simulink model "controller_ballcatcher"  (R2018b)
settings: Solver=FixedStepDiscrete  StartTime=0.0  StopTime=10.0  FixedStep=timing.T_iiwa  RelTol=1e-3
InitFcn:
  | iiwa_joint_trajectoryfollowingcontrol_rigid_parameters;
values from neighbouring files (symbols this model uses):
  filter_tau_p_slow_T_1 = filter_tau_slow_T_1    [parameters.m]
  filter_tau_p_T_1 = filter_tau_T_1    [parameters.m]
  filter_tau_slow_T_1 = 1./(2*pi*[200;200;200;200;200;200;200])    [parameters.m]
  filter_tau_T_1 = 1./(2*pi*[400;400;400;400;500;1000;1000])    [parameters.m]
  filter_theta_p_slow_T_1 = filter_tau_slow_T_1    [parameters.m]
  filter_theta_p_T_1 = filter_tau_T_1    [parameters.m]
  filter_theta_slow_T_1 = filter_tau_slow_T_1    [parameters.m]
  param_nullspace = struct()    [parameters.m]
  param_robot = struct()    [parameters.m]
  sensor_torque_offset = [0.53;-0.095;-0.189;0.07;-0.058;0.0025;-0.12]    [parameters.m]
  timing = struct()    [parameters.m]
undefined symbols (not defined in the file or in its folder): param_controller
settings Model: TCT_ExtModeMexArgs=[128 131 86 77 1 1],16842784  SimulationMode=external  Creator=cha  LastModifiedBy=stefanschweng
settings SolverCC: AutoInsertRateTranBlk=on
settings DataIOCC: LoggingToFile=on  LoggingFileName=benniii.mat
settings OptimizationCC: UseFloatMulNetSlope=on  PassReuseOutputArgsThreshold=0  LocalBlockOutputs=off  EfficientFloat2IntCast=on  OptimizeBlockOrder=speed  DifferentSizesBufferReuse=on
settings DebuggingCC: ParameterTunabilityLossMsg=error
settings HardwareCC: ProdLongLongMode=on
settings ModelReferenceCC: EnableParallelModelReferenceBuilds=on  ModelReferenceNumInstancesAllowed=Single
settings SFSimCC: SimUseLocalCustomCode=off  MATLABDynamicMemAlloc=off
settings RTWCC: Description=TwinCAT Target  SystemTargetFile=TwinCAT.tlc  GenCodeOnly=on  MakeCommand=make_tct  TemplateMakefile=tct_msbuild.tmf  GenerateReport=on  RTWUseLocalCustomCode=off  TargetLang=C++
settings RTWCC: CustomHeaderCode=|
  | #define fflush(stdout)
  | #define printf(...) m_spSrv->TcReportLog(ADSLOG_MSGTYPE_LOG,__VA_ARGS__)
settings CodeAppCC: ForceParamTrailComments=on  MaxIdLength=47  OperatorAnnotations=on  StateflowObjectComments=on  MATLABSourceComments=on
settings STFCustomTargetCC: TargetLangStandard=C++03 (ISO)  CompOptLevelCompliant=on  MATLABClassNameForMDSCustomization=Simulink.SoftwareTarget.TargetSpecificTriggerConfigurationBase  GRTInterface=on  SystemTargetFile=TwinCAT.tlc

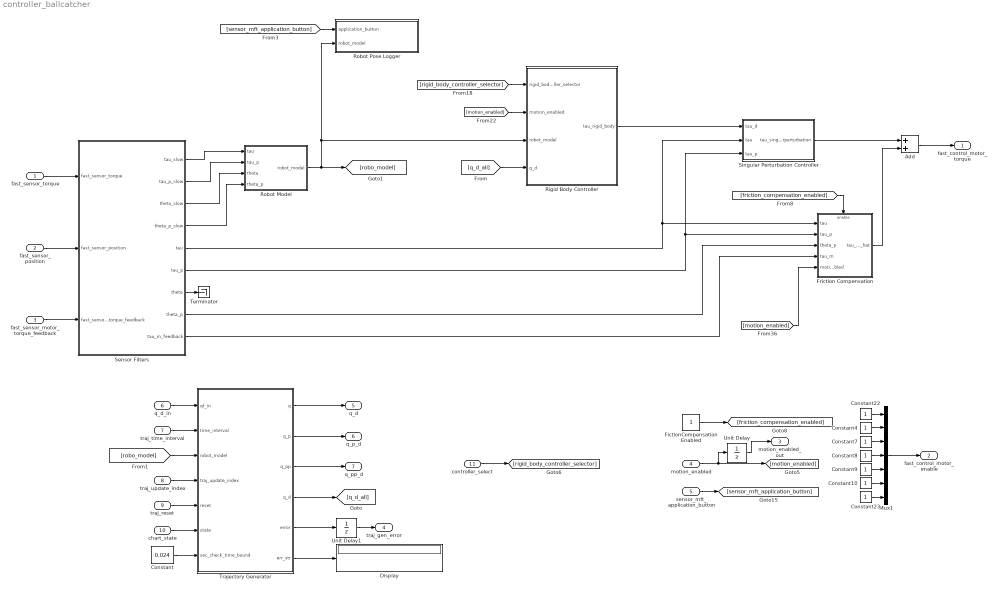
== system controller_ballcatcher ==
  fast_sensor_torque : Inport
  fast_sensor_position : Inport  Port=2
  fast_sensor_motor_torque_feedback : Inport  Port=3
  motion_enabled : Inport  Port=4
  sensor_mft_application_button : Inport  Port=5
  q_d_in : Inport  Port=6  PortDimensions=7
  traj_time_interval : Inport  Port=7  PortDimensions=2
  traj_update_index : Inport  Port=8
  traj_reset : Inport  Port=9
  chart_state : Inport  Port=10
  controller_select : Inport  Port=11
  Add : Sum
  Constant : Constant  Value=0.024
  Constant{4,7..10,22..23} (7 alike) : Constant
  Display : Display
  FictionCompensationEnabled : Constant
  Friction Compensation : Subsystem
  Mux1 : Mux  Inputs=7
  Rigid Body Controller : Subsystem
  Robot Model : MATLAB Function  TreatAsAtomicUnit=on
  Robot Pose Logger : MATLAB Function  TreatAsAtomicUnit=on
  Sensor Filters : Subsystem
  Singular Perturbation Controller : MATLAB Function  TreatAsAtomicUnit=on
  Terminator : Terminator
  Trajectory Generator : MATLAB Function  TreatAsAtomicUnit=on
  Unit Delay : UnitDelay  SampleTime=-1  HasFrameUpgradeWarning=on
  Unit Delay1 : UnitDelay  SampleTime=-1  HasFrameUpgradeWarning=on
  fast_control_motor_torque : Outport  VectorParamsAs1DForOutWhenUnconnected=off
  fast_control_motor_enable : Outport  Port=2  VectorParamsAs1DForOutWhenUnconnected=off
  motion_enabled_out : Outport  Port=3  VectorParamsAs1DForOutWhenUnconnected=off
  traj_gen_error : Outport  Port=4  OutDataTypeStr=boolean  VectorParamsAs1DForOutWhenUnconnected=off
  q_d : Outport  Port=5
  q_p_d : Outport  Port=6
  q_pp_d : Outport  Port=7
  wires:
  motion_enabled/1 -> Unit Delay/1, [motion_enabled]
  Sensor Filters/5(tau) -> Friction Compensation/1(tau), Singular Perturbation Controller/2(tau)
  Mux1/1 -> fast_control_motor_enable/1
  Constant22/1 -> Mux1/1
  Constant4/1 -> Mux1/2
  Constant7/1 -> Mux1/3
  Constant8/1 -> Mux1/4
  Constant9/1 -> Mux1/5
  Constant10/1 -> Mux1/6
  Constant23/1 -> Mux1/7
  fast_sensor_torque/1 -> Sensor Filters/1(fast_sensor_torque)
  fast_sensor_position/1 -> Sensor Filters/2(fast_sensor_position)
  fast_sensor_motor_torque_feedback/1 -> Sensor Filters/3(fast_sensor_motor_torque_feedback)
  Sensor Filters/9(tau_m_feedback) -> Friction Compensation/4(tau_m)
  Sensor Filters/6(tau_p) -> Friction Compensation/2(tau_p), Singular Perturbation Controller/3(tau_p)
  Sensor Filters/8(theta_p) -> Friction Compensation/3(theta_p)
  Friction Compensation/1(tau_fm_hat) -> Add/2
  [motion_enabled] -> Friction Compensation/5(motion_enabled)
  FictionCompensationEnabled/1 -> [friction_compensation_enabled]
  [friction_compensation_enabled] -> Friction Compensation/Enable
  Sensor Filters/7(theta) -> Terminator/1
  sensor_mft_application_button/1 -> [sensor_mft_application_button]
  Sensor Filters/1(tau_slow) -> Robot Model/1(tau)
  Sensor Filters/2(tau_p_slow) -> Robot Model/2(tau_p)
  Sensor Filters/3(theta_slow) -> Robot Model/3(theta)
  Sensor Filters/4(theta_p_slow) -> Robot Model/4(theta_p)
  [sensor_mft_application_button] -> Robot Pose Logger/1(application_button)
  Robot Model/1(robot_model) -> [robo_model], Rigid Body Controller/3(robot_model), Robot Pose Logger/2(robot_model)
  [rigid_body_controller_selector] -> Rigid Body Controller/1(rigid_body_controller_selector)
  [motion_enabled] -> Rigid Body Controller/2(motion_enabled)
  Singular Perturbation Controller/1(tau_singularperturbation) -> Add/1
  Rigid Body Controller/1(tau_rigid_body) -> Singular Perturbation Controller/1(tau_d)
  [q_d_all] -> Rigid Body Controller/4(q_d)
  Add/1 -> fast_control_motor_torque/1
  Unit Delay/1 -> motion_enabled_out/1
  Trajectory Generator/5(error) -> Unit Delay1/1
  Unit Delay1/1 -> traj_gen_error/1
  Trajectory Generator/3(q_pp) -> q_pp_d/1
  Trajectory Generator/2(q_p) -> q_p_d/1
  Trajectory Generator/1(q) -> q_d/1
  Trajectory Generator/4(q_d) -> [q_d_all]
  q_d_in/1 -> Trajectory Generator/1(qf_in)
  traj_time_interval/1 -> Trajectory Generator/2(time_interval)
  [robo_model] -> Trajectory Generator/3(robot_model)
  traj_update_index/1 -> Trajectory Generator/4(traj_update_index)
  traj_reset/1 -> Trajectory Generator/5(reset)
  chart_state/1 -> Trajectory Generator/6(state)
  controller_select/1 -> [rigid_body_controller_selector]
  Constant/1 -> Trajectory Generator/7(sec_check_time_bound)
  Trajectory Generator/6(err_str) -> Display/1

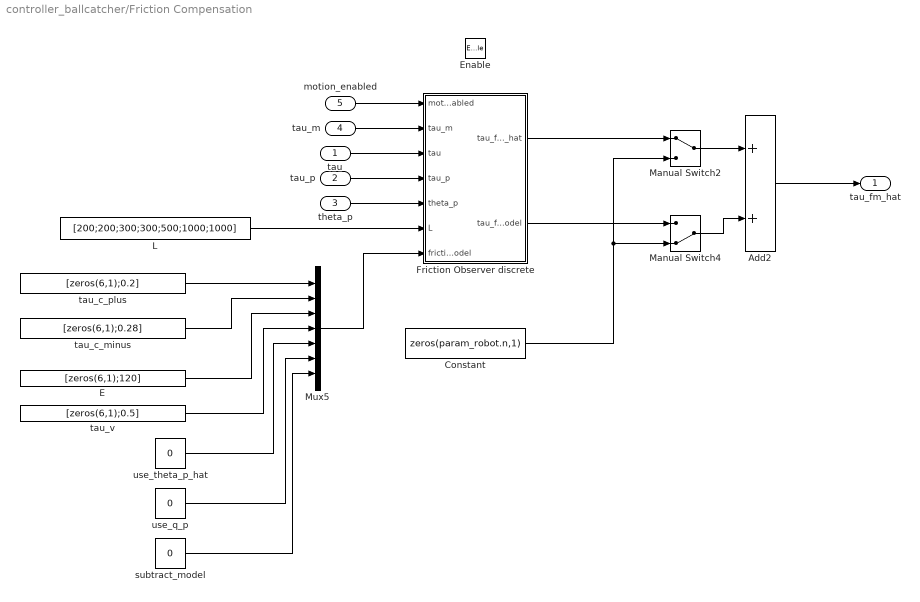
== system controller_ballcatcher/Friction Compensation ==
  tau : Inport
  tau_p : Inport  Port=2
  theta_p : Inport  Port=3
  tau_m : Inport  Port=4
  motion_enabled : Inport  Port=5
  Enable : EnablePort
  Add2 : Sum
  Constant : Constant  Value=zeros(param_robot.n,1)
  E : Constant  Value=[zeros(6,1);120]
  Friction Observer discrete : MATLAB Function  TreatAsAtomicUnit=on
  L : Constant  Value=[200;200;300;300;500;1000;1000]
  Manual Switch2 : ManualSwitch
  Manual Switch4 : ManualSwitch  CurrentSetting=0
  Mux5 : Mux  Inputs=7
  subtract_model : Constant  Value=0
  tau_c_minus : Constant  Value=[zeros(6,1);0.28]
  tau_c_plus : Constant  Value=[zeros(6,1);0.2]
  tau_v : Constant  Value=[zeros(6,1);0.5]
  use_q_p : Constant  Value=0
  use_theta_p_hat : Constant  Value=0
  tau_fm_hat : Outport  VectorParamsAs1DForOutWhenUnconnected=off
  wires:
  tau_p/1 -> Friction Observer discrete/4(tau_p)
  L/1 -> Friction Observer discrete/6(L)
  subtract_model/1 -> Mux5/7
  Friction Observer discrete/2(tau_f_model) -> Manual Switch4/1
  Manual Switch2/1 -> Add2/1
  tau_m/1 -> Friction Observer discrete/2(tau_m)
  use_q_p/1 -> Mux5/6
  Manual Switch4/1 -> Add2/2
  Friction Observer discrete/1(tau_fm_hat) -> Manual Switch2/1
  tau_c_minus/1 -> Mux5/2
  tau_v/1 -> Mux5/4
  use_theta_p_hat/1 -> Mux5/5
  Add2/1 -> tau_fm_hat/1
  Mux5/1 -> Friction Observer discrete/7(friction_model)
  motion_enabled/1 -> Friction Observer discrete/1(motion_enabled)
  tau_c_plus/1 -> Mux5/1
  theta_p/1 -> Friction Observer discrete/5(theta_p)
  Constant/1 -> Manual Switch4/2, Manual Switch2/2
  tau/1 -> Friction Observer discrete/3(tau)
  E/1 -> Mux5/3

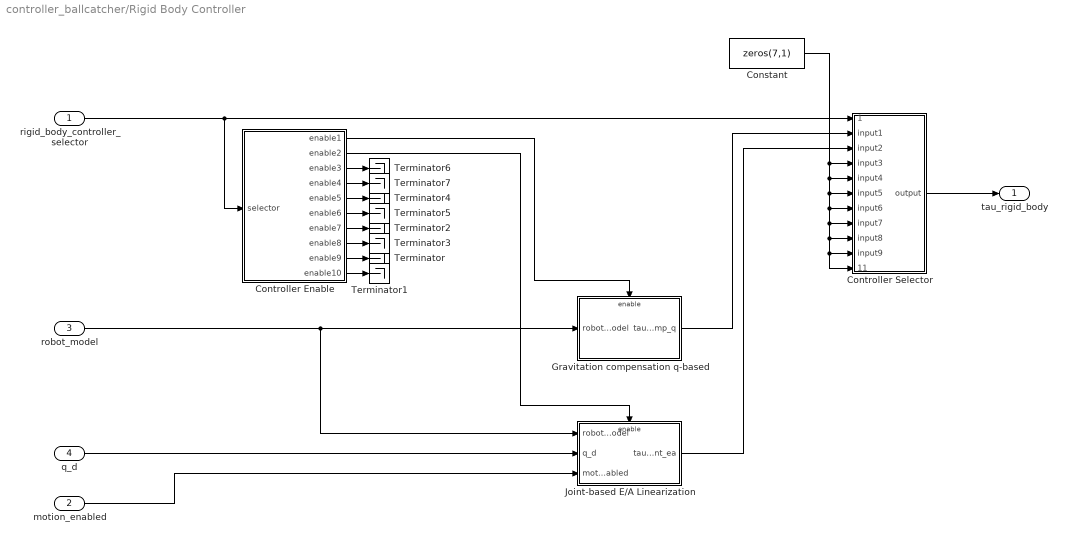
== system controller_ballcatcher/Rigid Body Controller ==
  rigid_body_controller_selector : Inport
  motion_enabled : Inport  Port=2
  robot_model : Inport  Port=3
  q_d : Inport  Port=4
  Constant : Constant  Value=zeros(7,1)
  Controller Enable : MATLAB Function  TreatAsAtomicUnit=on
  Controller Selector : MATLAB Function  TreatAsAtomicUnit=on
  Gravitation compensation q-based : Subsystem
  Joint-based E/A Linearization : Subsystem
  Terminator{,1..7} (8 alike) : Terminator
  tau_rigid_body : Outport  VectorParamsAs1DForOutWhenUnconnected=off
  wires:
  Controller Selector/1(output) -> tau_rigid_body/1
  rigid_body_controller_selector/1 -> Controller Selector/1(selector), Controller Enable/1(selector)
  robot_model/1 -> Gravitation compensation q-based/1(robot_model), Joint-based E/A Linearization/1(robot_model)
  Gravitation compensation q-based/1(tau_d_gravcomp_q) -> Controller Selector/2(input1)
  Controller Enable/1(enable1) -> Gravitation compensation q-based/Enable
  q_d/1 -> Joint-based E/A Linearization/2(q_d)
  motion_enabled/1 -> Joint-based E/A Linearization/3(motion_enabled)
  Joint-based E/A Linearization/1(tau_d_joint_ea) -> Controller Selector/3(input2)
  Controller Enable/2(enable2) -> Joint-based E/A Linearization/Enable
  Controller Enable/9(enable9) -> Terminator/1
  Controller Enable/10(enable10) -> Terminator1/1
  Controller Enable/7(enable7) -> Terminator2/1
  Controller Enable/8(enable8) -> Terminator3/1
  Controller Enable/6(enable6) -> Terminator5/1
  Controller Enable/4(enable4) -> Terminator7/1
  Controller Enable/5(enable5) -> Terminator4/1
  Constant/1 -> Controller Selector/4(input3), Controller Selector/11(input10), Controller Selector/10(input9), Controller Selector/9(input8), Controller Selector/8(input7), Controller Selector/7(input6), Controller Selector/6(input5), Controller Selector/5(input4)
  Controller Enable/3(enable3) -> Terminator6/1

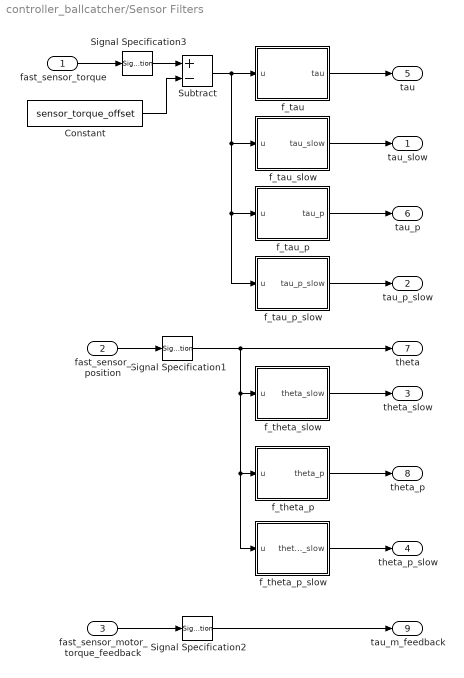
== system controller_ballcatcher/Sensor Filters ==
  fast_sensor_torque : Inport
  fast_sensor_position : Inport  Port=2
  fast_sensor_motor_torque_feedback : Inport  Port=3
  Constant : Constant  Value=sensor_torque_offset
  Signal Specification1 : SignalSpecification  Dimensions=7
  Signal Specification2 : SignalSpecification  Dimensions=7
  Signal Specification3 : SignalSpecification  Dimensions=7
  Subtract : Sum  Inputs=+-
  f_tau : MATLAB Function  TreatAsAtomicUnit=on
  f_tau_p : MATLAB Function  TreatAsAtomicUnit=on
  f_tau_p_slow : MATLAB Function  TreatAsAtomicUnit=on
  f_tau_slow : MATLAB Function  TreatAsAtomicUnit=on
  f_theta_p : MATLAB Function  TreatAsAtomicUnit=on
  f_theta_p_slow : MATLAB Function  TreatAsAtomicUnit=on
  f_theta_slow : MATLAB Function  TreatAsAtomicUnit=on
  tau_slow : Outport  VectorParamsAs1DForOutWhenUnconnected=off
  tau_p_slow : Outport  Port=2  VectorParamsAs1DForOutWhenUnconnected=off
  theta_slow : Outport  Port=3  VectorParamsAs1DForOutWhenUnconnected=off
  theta_p_slow : Outport  Port=4  VectorParamsAs1DForOutWhenUnconnected=off
  tau : Outport  Port=5  VectorParamsAs1DForOutWhenUnconnected=off
  tau_p : Outport  Port=6  VectorParamsAs1DForOutWhenUnconnected=off
  theta : Outport  Port=7  VectorParamsAs1DForOutWhenUnconnected=off
  theta_p : Outport  Port=8  VectorParamsAs1DForOutWhenUnconnected=off
  tau_m_feedback : Outport  Port=9  VectorParamsAs1DForOutWhenUnconnected=off
  wires:
  fast_sensor_position/1 -> Signal Specification1/1
  fast_sensor_motor_torque_feedback/1 -> Signal Specification2/1
  f_theta_p/1(theta_p) -> theta_p/1
  Signal Specification1/1 -> theta/1, f_theta_slow/1(u), f_theta_p_slow/1(u), f_theta_p/1(u)
  f_tau_p/1(tau_p) -> tau_p/1
  f_theta_p_slow/1(theta_p_slow) -> theta_p_slow/1
  f_tau/1(tau) -> tau/1
  Signal Specification2/1 -> tau_m_feedback/1
  f_theta_slow/1(theta_slow) -> theta_slow/1
  f_tau_slow/1(tau_slow) -> tau_slow/1
  f_tau_p_slow/1(tau_p_slow) -> tau_p_slow/1
  Constant/1 -> Subtract/2
  Subtract/1 -> f_tau/1(u), f_tau_slow/1(u), f_tau_p_slow/1(u), f_tau_p/1(u)
  fast_sensor_torque/1 -> Signal Specification3/1
  Signal Specification3/1 -> Subtract/1

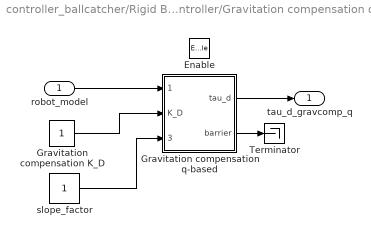
== system controller_ballcatcher/Rigid Body Controller/Gravitation compensation q-based ==
  robot_model : Inport
  Enable : EnablePort  StatesWhenEnabling=reset
  Gravitation compensation q-based : MATLAB Function  TreatAsAtomicUnit=on
  Gravitation compensation K_D : Constant
  Terminator : Terminator
  slope_factor : Constant
  tau_d_gravcomp_q : Outport  VectorParamsAs1DForOutWhenUnconnected=off
  wires:
  robot_model/1 -> Gravitation compensation q-based/1(robot_model)
  Gravitation compensation q-based/1(tau_d) -> tau_d_gravcomp_q/1
  Gravitation compensation K_D/1 -> Gravitation compensation q-based/2(K_D)
  Gravitation compensation q-based/2(barrier) -> Terminator/1
  slope_factor/1 -> Gravitation compensation q-based/3(slope_factor)

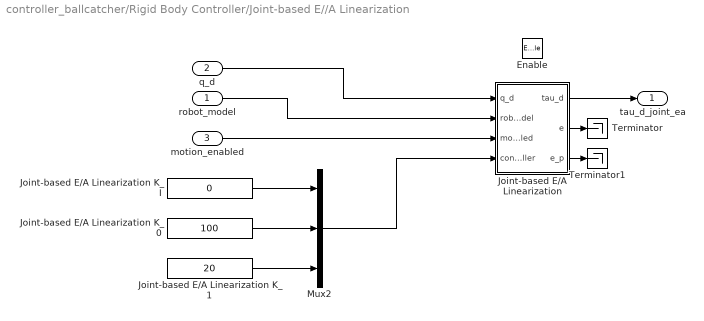
== system controller_ballcatcher/Rigid Body Controller/Joint-based E//A Linearization ==
  robot_model : Inport
  q_d : Inport  Port=2
  motion_enabled : Inport  Port=3
  Enable : EnablePort  StatesWhenEnabling=reset
  Joint-based E/A Linearization : MATLAB Function  TreatAsAtomicUnit=on
  Joint-based E/A Linearization K_0 : Constant  Value=100
  Joint-based E/A Linearization K_1 : Constant  Value=20
  Joint-based E/A Linearization K_I : Constant  Value=0
  Mux2 : Mux  Inputs=3
  Terminator : Terminator
  Terminator1 : Terminator
  tau_d_joint_ea : Outport  VectorParamsAs1DForOutWhenUnconnected=off
  wires:
  motion_enabled/1 -> Joint-based E/A Linearization/3(motion_enabled)
  Joint-based E/A Linearization K_I/1 -> Mux2/1
  Joint-based E/A Linearization K_1/1 -> Mux2/3
  Joint-based E/A Linearization K_0/1 -> Mux2/2
  Joint-based E/A Linearization/1(tau_d) -> tau_d_joint_ea/1
  q_d/1 -> Joint-based E/A Linearization/1(q_d)
  Mux2/1 -> Joint-based E/A Linearization/4(controller)
  robot_model/1 -> Joint-based E/A Linearization/2(robot_model)
  Joint-based E/A Linearization/2(e) -> Terminator/1
  Joint-based E/A Linearization/3(e_p) -> Terminator1/1

== matlab function controller_ballcatcher/Sensor Filters/f_tau ==
  data: u input; tau output; param_controller parameter; filter_tau_T_1 parameter
function tau = func(u,param_controller, filter_tau_T_1)
  persistent x;
  
  T_1=filter_tau_T_1;
  alpha=exp(-param_controller.T_a./T_1);
  if(isempty(x))
    x=1./(1-alpha).*u;
    tau=u;
  else
    tau=(1-alpha).*x;
    x=alpha.*x+u;
  end
end

== matlab function controller_ballcatcher/Sensor Filters/f_tau_p ==
  data: u input; tau_p output; filter_tau_p_T_1 parameter; param_controller parameter
function tau_p = func(u,filter_tau_p_T_1,param_controller)
  persistent x;
  
  T_1=filter_tau_p_T_1;
  V=1/param_controller.T_a*(1-exp(-param_controller.T_a./T_1));
  if(isempty(x))
    x=-V.*u;
    tau_p=zeros(size(u));
  else
    tau_p=x+V.*u;
    x=exp(-param_controller.T_a./T_1).*x+(exp(-param_controller.T_a./T_1)-1).*V.*u;
  end
end

== matlab function controller_ballcatcher/Singular Perturbation Controller ==
  data: tau_d input; tau input; tau_p input; tau_singularperturbation output; param_controller parameter
function tau_singularperturbation  = fcn(tau_d,tau,tau_p,param_controller)
  %Implementation is taken from Ott 2008, chapter 5.4.
  tau_singularperturbation_controller_K=-param_controller.singular_perturbation.K_tau.*(tau-tau_d);
  tau_singularperturbation_controller_D=-param_controller.singular_perturbation.D_tau.*tau_p;
  tau_singularperturbation_controller=tau_singularperturbation_controller_K...
    +tau_singularperturbation_controller_D;
  tau_singularperturbation=tau_d+tau_singularperturbation_controller;
end

== matlab function controller_ballcatcher/Trajectory Generator ==
  data: q output; qf_in input size=7; time_interval input; q_p output; q_pp output; param_robot parameter; q_d output; robot_model input; traj_update_index input; timing parameter; reset input; state input; error output size=1; sec_check_time_bound input; err_str output
function [q,q_p,q_pp,q_d,error,err_str]  = fcn(qf_in,time_interval,param_robot,robot_model,traj_update_index,timing,reset,state,sec_check_time_bound)
    persistent q0 q0_p q0_pp qf T_0 T_f q_ q_p_ q_pp_ t_ started error_ traj_update_index_last error_num;
    
    n = 7;
    qf_p = zeros(n,1);
    qf_pp = zeros(n,1);
    
    if isempty(q0)
      q0 = robot_model.q;
      q0_p = zeros(n,1);
      q0_pp = zeros(n,1);
      qf = robot_model.q;
      T_0 = 0;
      T_f = 0;
      q_ = robot_model.q;
      q_p_ = zeros(n,1);
      q_pp_ = zeros(n,1);
      t_ = 0;
      started = false;
      error_ = false;
      error_num = 0;
      traj_update_index_last = 0;
    end
    
    if (traj_update_index_last ~= traj_update_index) || reset
       q0 = q_;
       q0_p = q_p_;
       q0_pp = q_pp_;
        
       if reset
         qf = robot_model.q;
         T_0 = 0;
         T_f = 0;
         started = false;
       else
         qf = qf_in;
         T_0 = time_interval(1);
         T_f = time_interval(2);
         started = true;
       end
       
       t_ = 0;
    end
    
    if reset
      error_ = false;
      error_num = 0;
    end
    
    T = T_f-T_0;
    
    H = robot_model.H;
    x_ee = H(1,4);
    y_ee = H(2,4);
    z_ee = H(3,4);
    
    % safety check: check if EE moves to far from starting position
    if (state == 2 && (x_ee < 0.2 || abs(y_ee) > 0.5 || z_ee > 1))
      error_ = true;
      error_num = -1;
      started = false;
      fprintf('Error in Trajectory Generation: Endeffector out of operational space.');
    end
    
    if error_
        started = false;
    elseif t_ < 0
        started = false;
        q_d_temp=[q0;zeros(size(q0));zeros(size(q0))];
        q_ = q_d_temp(1:7);
        q_p_ = q_d_temp(8:14);
        q_pp_ = q_d_temp(15:21);
    elseif(t_>=T)
        started = false;
        q_d_temp=[qf;zeros(size(qf));zeros(size(qf))];
        q_ = q_d_temp(1:7);
        q_p_ = q_d_temp(8:14);
        q_pp_ = q_d_temp(15:21);
    elseif started
        t0 = 0;
        tf = T;

        for i = 1:n
            A = [1,t0,(t0^2)/2,(t0^3)/6,(t0^4)/24,(t0^5)/120;...
                1,tf,(tf^2)/2,(tf^3)/6,(tf^4)/24,(tf^5)/120;...
                0,1,t0,(t0^2)/2,(t0^3)/6,(t0^4)/24;...
                0,1,tf,(tf^2)/2,(tf^3)/6,(tf^4)/24;...
                0,0,1,t0,(t0^2)/2,(t0^3)/6;...
                0,0,1,tf,(tf^2)/2,(tf^3)/6];

            coeffs = (A\[q0(i);qf(i);q0_p(i);qf_p(i);q0_pp(i);qf_pp(i)])';
            
            p = flip(coeffs);
            % take factorials into account to match initial equations
            p(1) = p(1)/120;
            p(2) = p(2)/24;
            p(3) = p(3)/6;
            p(4) = p(4)/2;
            
            q_(i) = polyval(p,t_);
            
            pd = polyder(p);
            q_p_(i) = polyval(pd,t_);
            
            pdd = polyder(pd);
            q_pp_(i) = polyval(pdd,t_);
            
            % safety check: check if q_p exceeds velocity limits
            t0_check = t0;
            if state ~= 2
                t0_check = t_;
            end
            
            tf_check = t0_check+sec_check_time_bound;
            if tf_check > tf
               tf_check = tf; 
            end
            
            % check interval limits
            if abs(polyval(pd,t0_check)) >= param_robot.q_p_limit_upper(i) ||...
                    abs(polyval(pd,tf_check)) >= param_robot.q_p_limit_upper(i)
                error_ = true;
                started = false;
                fprintf('Error in Trajectory Generation: Planned trajectory exceeds joint velocitiy limits in Axis %i', int8(i));
                error_num = i;
                break;
            end
            
            % check extremas within the time interval
            q_pp_roots = roots(pdd);
            q_p_extrema = polyval(pd,q_pp_roots);
            pddd = polyder(pdd);

            for z=1:size(q_p_extrema,1)
              if polyval(pddd,q_pp_roots(z))~=0 &&...
                  q_pp_roots(z)<=(t0_check+sec_check_time_bound) &&...
                  q_pp_roots(z)>=t0_check &&...
                  (q_p_extrema(z)>=param_robot.q_p_limit_upper(i) ||...
                  q_p_extrema(z)<=param_robot.q_p_limit_lower(i))
                error_ = true;
                started = false;
                fprintf('Error in Trajectory Generation: Planned trajectory exceeds joint velocitiy limits in Axis %i', int8(i));
                error_num = i;
                break;
              end
            end
        end    
    end
    
    q = q_;
    q_p = q_p_;
    q_pp = q_pp_;
    
    q_d = zeros(3*n,1);
    q_d(1:n)=q;
    q_d(n+1:2*n)=q_p;
    q_d(2*n+1:3*n)=q_pp;
    
    if started
      if state==2
        t_ = t_ + (timing.T_iiwa);
      else
        t_ = t_ + timing.T_iiwa;
      end 
    else
        %Hold last position, set velocity and acceleration zero
        q_d(n+1:end)=0;
    end
    
    error = error_;
    err_str = error_num;
    
    q = rad2deg(q);
    q_p = rad2deg(q_p);
    q_pp = rad2deg(q_pp);
    
    traj_update_index_last = traj_update_index;

== matlab function controller_ballcatcher/Robot Pose Logger ==
  data: application_button input; robot_model input
function fcn(application_button,robot_model)
  persistent last_application_button;

  if(isempty(last_application_button))
    last_application_button=application_button;
  end
  
  if(last_application_button~=application_button && application_button)
    fprintf('[%.10f,%.10f,%.10f,%.10f;%.10f,%.10f,%.10f,%.10f;%.10f,%.10f,%.10f,%.10f],...',...
      robot_model.H(1,1),robot_model.H(1,2),robot_model.H(1,3),robot_model.H(1,4),...
      robot_model.H(2,1),robot_model.H(2,2),robot_model.H(2,3),robot_model.H(2,4),...
      robot_model.H(3,1),robot_model.H(3,2),robot_model.H(3,3),robot_model.H(3,4));
  end
  
  last_application_button=application_button;
end

== matlab function controller_ballcatcher/Sensor Filters/f_tau_slow ==
  data: u input; tau_slow output; param_controller parameter; filter_tau_slow_T_1 parameter
function tau_slow = func(u,param_controller, filter_tau_slow_T_1)
  persistent x;
  
  T_1=filter_tau_slow_T_1;
  alpha=exp(-param_controller.T_a./T_1);
  if(isempty(x))
    x=1./(1-alpha).*u;
    tau_slow=u;
  else
    tau_slow=(1-alpha).*x;
    x=alpha.*x+u;
  end
end

== matlab function controller_ballcatcher/Rigid Body Controller/Gravitation compensation q-based/Gravitation compensation q-based ==
  data: robot_model input; tau_d output; K_D input; slope_factor input; param_nullspace parameter; barrier output; param_robot parameter
function [tau_d,barrier] = fcn(robot_model, K_D,slope_factor,param_nullspace,param_robot)
  n=param_robot.n;
  %% Barrier or penalty functions for nullspace controller
  %Desired position for nullspace
  p_1=...
    slope_factor*param_nullspace.q_limit_slope(1:n)./...
      (1./(param_nullspace.q_limit_range(1:n).^2)...
      -1./((param_nullspace.q_limit_upper(1:n)-param_nullspace.q_limit_lower(1:n)-param_nullspace.q_limit_range(1:n)).^2));
    
  q=robot_model.q;
  barrier=zeros(size(q));
  valid=q<param_nullspace.q_limit_upper(1:n) & q>param_nullspace.q_limit_lower(1:n);
  inside=q<(param_nullspace.q_limit_upper(1:n)-param_nullspace.q_limit_range(1:n)) & ...
    q>(param_nullspace.q_limit_lower(1:n)+param_nullspace.q_limit_range(1:n));
  barrier(valid)=(1./(q(valid)-param_nullspace.q_limit_upper(valid)).^2 ...
      -1./(param_nullspace.q_limit_lower(valid)-q(valid)).^2).*p_1(valid)...
    -slope_factor*param_nullspace.q_limit_slope(valid).*sign(q(valid));
  barrier(~valid)=NaN;
  barrier(inside)=0;
  
  tau_d=robot_model.g-K_D*robot_model.q_p-barrier;
end

== matlab function controller_ballcatcher/Sensor Filters/f_theta_p ==
  data: u input; theta_p output; filter_theta_p_T_1 parameter; param_controller parameter
function theta_p = func(u,filter_theta_p_T_1,param_controller)
  persistent x;
  
  T_1=filter_theta_p_T_1;
  V=1/param_controller.T_a*(1-exp(-param_controller.T_a./T_1));
  if(isempty(x))
    x=-V.*u;
    theta_p=zeros(size(u));
  else
    theta_p=x+V.*u;
    x=exp(-param_controller.T_a./T_1).*x+(exp(-param_controller.T_a./T_1)-1).*V.*u;
  end
end

== matlab function controller_ballcatcher/Rigid Body Controller/Joint-based E//A Linearization/Joint-based E//A Linearization ==
  data: q_d input; robot_model input; motion_enabled input; tau_d output; param_robot parameter; controller input; param_controller parameter; e output; e_p output
function [tau_d,e,e_p] = fcn(q_d,robot_model,motion_enabled, param_robot,controller,param_controller)
  persistent e_I;
  
  if(~motion_enabled || isempty(e_I))
    e_I=zeros(param_robot.n,1);
  end
  
  q_pp_d=q_d(2*param_robot.n+1:3*param_robot.n);
  q_p_d=q_d(param_robot.n+1:2*param_robot.n);
  q_d=q_d(1:param_robot.n);
  
  K_I=controller(1)*ones(param_robot.n,1);
  K_0=controller(2)*ones(param_robot.n,1);
  K_1=controller(3)*ones(param_robot.n,1);
  
  q=robot_model.q;
  q_p=robot_model.q_p;
  
  %Common "Computed Torque" equations
  M=robot_model.M;
  C=robot_model.C;
  g=robot_model.g;
  n=C*q_p+g;

  e=q-q_d;
  e_p=q_p-q_p_d;
  v=q_pp_d-K_1.*e_p-K_0.*e-K_I.*e_I;
  
  tau_d=M*v+n;
  
  e_I=e_I+e*param_controller.T_a;
end

== matlab function controller_ballcatcher/Robot Model ==
  data: tau input; tau_p input; theta input; robot_model output Bus: robot_model; theta_p input; param_robot parameter; param_controller parameter
function robot_model = fcn(tau,tau_p,theta,theta_p,param_robot,param_controller)
  K=param_robot.K;
  
  robot_model=struct();
  %The calculation of q and q_p has to be performed with consistent cutoff
  %frequencies for the corresponding filters. The filters for q, q_p, tau
  %and tau_p have to have the same cutoff frequency.
  q=theta-diag(K).\tau;
  q_p=theta_p-diag(K).\tau_p;
  robot_model.q=q;
  robot_model.q_p=q_p;
  %Path Following Control with reverse kinematic
  robot_model.H=[iiwa_homogeneous_transformation_endeffector(q,param_robot);[0 0 0 1]];
  robot_model.J=iiwa_jacobian(q,param_robot);
  robot_model.J_p=iiwa_jacobian_p(q,q_p,param_robot);
  %If the singular perturbation controller is selected, the mass matrix has
  %to be modified according to Ott2008, Eq. (5.28).
  robot_model.M=iiwa_reduced_inertia_matrix(q,param_robot);
  %More efficient implementation for M+(I+K_tau)\B with diagonal
  %matrices K_tau and B: Only handle the diagonal elements.
  robot_model.M=robot_model.M+diag((1+param_controller.singular_perturbation.K_tau).\diag(param_robot.B));
  robot_model.C=iiwa_reduced_coriolis_matrix(q,q_p,param_robot);
  robot_model.g=iiwa_gravitational_force(q,param_robot);
end

== matlab function controller_ballcatcher/Friction Compensation/Friction Observer discrete ==
  settings: sampleTime=param.T_a
  data: motion_enabled input; tau_m input; tau input; tau_p input; theta_p input; tau_fm_hat output; param_robot parameter; L input; param_controller parameter; tau_f_model output; friction_model input
function [tau_fm_hat,tau_f_model]  = fcn(motion_enabled,tau_m,tau,tau_p,theta_p, param_robot,L, param_controller, friction_model)
  persistent x_theta_p_hat;
  
  T_a=param_controller.T_a;
  B=param_robot.B;

  if(isempty(x_theta_p_hat))
    x_theta_p_hat=zeros(param_robot.n,1);
  end
  
  if(motion_enabled)
    tau_c_plus=friction_model(1:param_robot.n);
    tau_c_minus=friction_model(param_robot.n+1:2*param_robot.n);
    E=friction_model(2*param_robot.n+1:3*param_robot.n);
    tau_v=friction_model(3*param_robot.n+1:4*param_robot.n);
    use_theta_p_hat=friction_model(4*param_robot.n+1);
    use_q_p=friction_model(4*param_robot.n+2);
    subtract_model=friction_model(4*param_robot.n+3);
    if(use_theta_p_hat)
      tmp=x_theta_p_hat;
    else
      tmp=theta_p;
    end
    if(use_q_p)
      q_p=tmp-param_robot.K\tau_p;
    else
      q_p=tmp;
    end
    %tau_f_model is the downforce friction, which cannot be observed, since
    %it happens after the torque sensor with respect to q_p.
    %This friction torque can be added to the motor torque to compensate for
    %this additional friction. It is _not_ subtracted from tau_m in the
    %friction observer, since it is additional torque, which has to appear
    %at the torque sensor and is required to overcome friction in the
    %downforce train.
    tau_f_model=zeros(size(q_p));
    c=q_p>=0;
    tau_f_model(c)=tau_c_plus(c).*tanh(E(c).*q_p(c));
    tau_f_model(~c)=tau_c_minus(~c).*tanh(E(~c).*q_p(~c));
    tau_f_model=tau_f_model+tau_v.*q_p;
    
    %Estimated, unmodeled friction
    tau_fm_hat=-L.*diag(param_robot.B).*(theta_p-x_theta_p_hat);
    %The term tau_m is the feedback torque from the motor. It contains the
    %added "tau_fm_hat", therefore it has to be subtracted, before feeding
    %it into the observer.
    %Notice, that not the actual control value is used, but the sensor
    %value from the motor. The latter signal is very, very noisy (standard
    %deviation of about 3 Nm at rest), but it shows the best behaviour for
    %estimating friction. It is also convenient, that the sensor value
    %implicitly contains the low-level saturation of the commanded value.
    if(subtract_model)
      x_theta_p_hat=x_theta_p_hat+T_a*(B\(tau_m-tau-tau_f_model-tau_fm_hat));
    else
      x_theta_p_hat=x_theta_p_hat+T_a*(B\(tau_m-tau-tau_fm_hat));
    end
  else
    x_theta_p_hat=zeros(param_robot.n,1);
    tau_fm_hat=zeros(param_robot.n,1);
    tau_f_model=zeros(param_robot.n,1);
  end
end

== matlab function controller_ballcatcher/Sensor Filters/f_theta_slow ==
  data: u input; theta_slow output; param_controller parameter; filter_theta_slow_T_1 parameter
function theta_slow = func(u,param_controller, filter_theta_slow_T_1)
  persistent x;
  
  T_1=filter_theta_slow_T_1;
  alpha=exp(-param_controller.T_a./T_1);
  if(isempty(x))
    x=1./(1-alpha).*u;
    theta_slow=u;
  else
    theta_slow=(1-alpha).*x;
    x=alpha.*x+u;
  end
end

== matlab function controller_ballcatcher/Sensor Filters/f_tau_p_slow ==
  data: u input; tau_p_slow output; filter_tau_p_slow_T_1 parameter; param_controller parameter
function tau_p_slow = func(u,filter_tau_p_slow_T_1,param_controller)
  persistent x;
  
  T_1=filter_tau_p_slow_T_1;
  V=1/param_controller.T_a*(1-exp(-param_controller.T_a./T_1));
  if(isempty(x))
    x=-V.*u;
    tau_p_slow=zeros(size(u));
  else
    tau_p_slow=x+V.*u;
    x=exp(-param_controller.T_a./T_1).*x+(exp(-param_controller.T_a./T_1)-1).*V.*u;
  end
end

== matlab function controller_ballcatcher/Sensor Filters/f_theta_p_slow ==
  data: u input; theta_p_slow output; filter_theta_p_slow_T_1 parameter; param_controller parameter
function theta_p_slow = func(u,filter_theta_p_slow_T_1,param_controller)
  persistent x;
  
  T_1=filter_theta_p_slow_T_1;
  V=1/param_controller.T_a*(1-exp(-param_controller.T_a./T_1));
  if(isempty(x))
    x=-V.*u;
    theta_p_slow=zeros(size(u));
  else
    theta_p_slow=x+V.*u;
    x=exp(-param_controller.T_a./T_1).*x+(exp(-param_controller.T_a./T_1)-1).*V.*u;
  end
end

== matlab function controller_ballcatcher/Rigid Body Controller/Controller Enable ==
  data: enable1 output; enable2 output; enable3 output; enable4 output; enable5 output; enable6 output; enable7 output; enable8 output; selector input uint32; enable9 output; enable10 output
function [enable1,enable2,enable3,enable4,enable5,enable6,enable7,enable8,enable9,enable10] = fcn(selector)
    enable1=(selector==1);
    enable2=(selector==2);
    enable3=(selector==3);
    enable4=(selector==4);
    enable5=(selector==5);
    enable6=(selector==6);
    enable7=(selector==7);
    enable8=(selector==8);
    enable9=(selector==9);
    enable10=(selector==10);
end

== matlab function controller_ballcatcher/Rigid Body Controller/Controller Selector ==
  data: selector input uint32; input1 input; input2 input; input3 input; input4 input; input5 input; input6 input; input7 input; input8 input; output output; input9 input; input10 input
function output = fcn(selector,input1,input2,input3,input4,input5,input6,input7,input8,input9,input10)
    switch selector
        case 1
            output=input1;
        case 2
            output=input2;
        case 3
            output=input3;
        case 4
            output=input4;
        case 5
            output=input5;
        case 6
            output=input6;
        case 7
            output=input7;
        case 8
            output=input8;
        case 9
            output=input9;
        case 10
            output=input10;
        otherwise
            output=zeros(size(input1));
    end
end
